simulink model "solution1_7009_newfmu"  (R2017b)
settings: Solver=FixedStepAuto  StartTime=0.0  StopTime=inf  FixedStep=0.01  RelTol=1e-3
values from neighbouring files (symbols this model uses):
  g = 9.81    [initialize_simplemodel.m]    (also in initialize_simplemodel_Trial.m; tire_friction_circle.m)
  h = 0.35    [initialize_simplemodel.m]    (also in initialize_simplemodel_Trial.m)
  lf = 1.4    [initialize_simplemodel.m]    (also in initialize_simplemodel_Trial.m)
  lr = 1.345    [initialize_simplemodel.m]    (also in initialize_simplemodel_Trial.m)
  m = 1400    [initialize_simplemodel.m]    (also in initialize_simplemodel_Trial.m = 1300; tire_friction_circle.m = 1300)
  r = 0.34    [initialize_simplemodel.m]    (also in initialize_simplemodel_Trial.m)
  tr = 1.684/2    (= 0.842)    [initialize_simplemodel.m]    (also in initialize_simplemodel_Trial.m)
  v_init = 60*5/18    (= 16.6666666667)    [initialize_simplemodel.m]    (also in initialize_simplemodel_Trial.m)
undefined symbols (not defined in the file or in its folder): DiscIntNeverNeededParam
libraries: simulink x28
(part 1 of 2)
settings Model: Creator=ashwin.ramanujam  LastModifiedBy=gandh
settings DataIOCC: SignalLogging=off

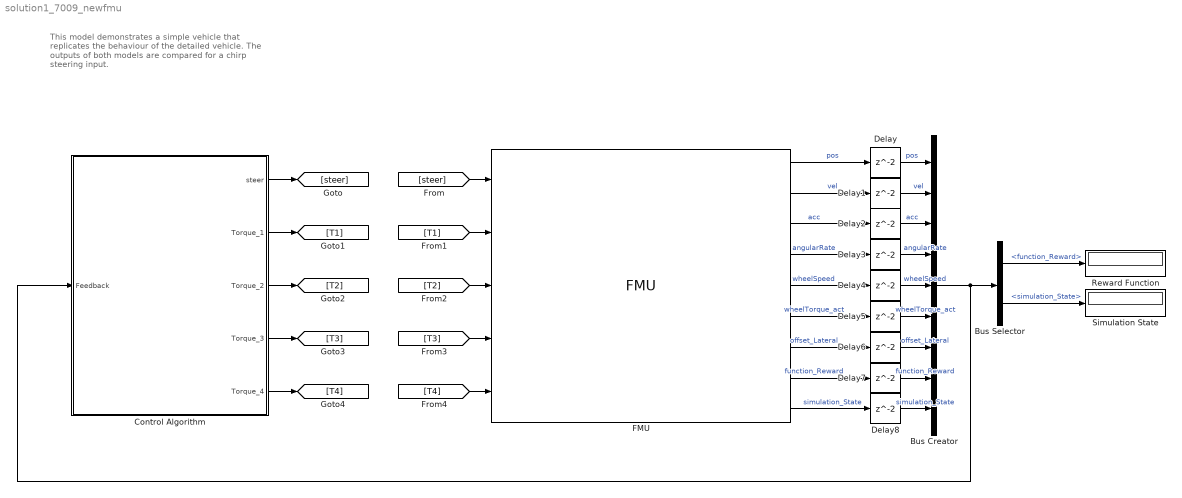
== system solution1_7009_newfmu ==
  note: This model demonstrates a simple vehicle that replicates the behaviour of the detailed vehicle. The outputs of both models are compared for a chirp steering input.
  Bus Creator : BusCreator  Inputs=9
  Bus Selector : BusSelector  OutputSignals=function_Reward,simulation_State
  Control Algorithm : Subsystem
  Delay{,1..8} (9 alike) : Delay
  FMU : FMU  FMUName=MED2018_VehicleModel_sclxversion.fmu  FMUMode=CoSimulation  FMUSampleTime=-1  mask(MED2018.VehicleModel [Co-Simulation, v2.0]){}
      mask Display:
      | disp('MED2018.VehicleModel');
      | port_label('output',1,'Position');
      | port_label('output',2,'Velocity');
      | port_label('output',3,'Acceleration');
      | port_label('output',4,'angularRate');
      | port_label('output',5,'wheelSpeed');
      | port_label('output',6,'wheelTorque_act');
      | port_label('output',7,'offset_Lateral');
      | port_label('output',8,'function_Reward');
      | port_label('output',9,'simulation_State');
      | port_label('input',1,'steering_Angle');
      | port_label('input',2,'wheelTorque_cmd_FL');
      | port_label('input',3,'wheelTorque_cmd_FR');
      | port_label('input',4,'wheelTorque_cmd_RL');
      | port_label('input',5,'wheelTorque_cmd_RR');
  Reward Function : Display
  Simulation State : Display
  wires:
  [steer] -> FMU/1
  [T4] -> FMU/5
  [T1] -> FMU/2
  [T2] -> FMU/3
  [T3] -> FMU/4
  Control Algorithm/1(steer) -> [steer]
  Control Algorithm/2(Torque_1) -> [T1]
  Control Algorithm/3(Torque_2) -> [T2]
  Control Algorithm/4(Torque_3) -> [T3]
  Control Algorithm/5(Torque_4) -> [T4]
  FMU/1 -> Delay/1  "pos"
  FMU/6 -> Delay5/1  "wheelTorque_act"
  FMU/8 -> Delay7/1  "function_Reward"
  FMU/3 -> Delay2/1  "acc"
  FMU/5 -> Delay4/1  "wheelSpeed"
  FMU/7 -> Delay6/1  "offset_Lateral"
  FMU/2 -> Delay1/1  "vel"
  FMU/4 -> Delay3/1  "angularRate"
  FMU/9 -> Delay8/1  "simulation_State"
  Bus Creator/1 -> Control Algorithm/1(Feedback), Bus Selector/1
  Bus Selector/1 -> Reward Function/1  "<function_Reward>"
  Bus Selector/2 -> Simulation State/1  "<simulation_State>"
  Delay/1 -> Bus Creator/1  "pos"
  Delay1/1 -> Bus Creator/2  "vel"
  Delay2/1 -> Bus Creator/3  "acc"
  Delay3/1 -> Bus Creator/4  "angularRate"
  Delay4/1 -> Bus Creator/5  "wheelSpeed"
  Delay5/1 -> Bus Creator/6  "wheelTorque_act"
  Delay6/1 -> Bus Creator/7  "offset_Lateral"
  Delay7/1 -> Bus Creator/8  "function_Reward"
  Delay8/1 -> Bus Creator/9  "simulation_State"

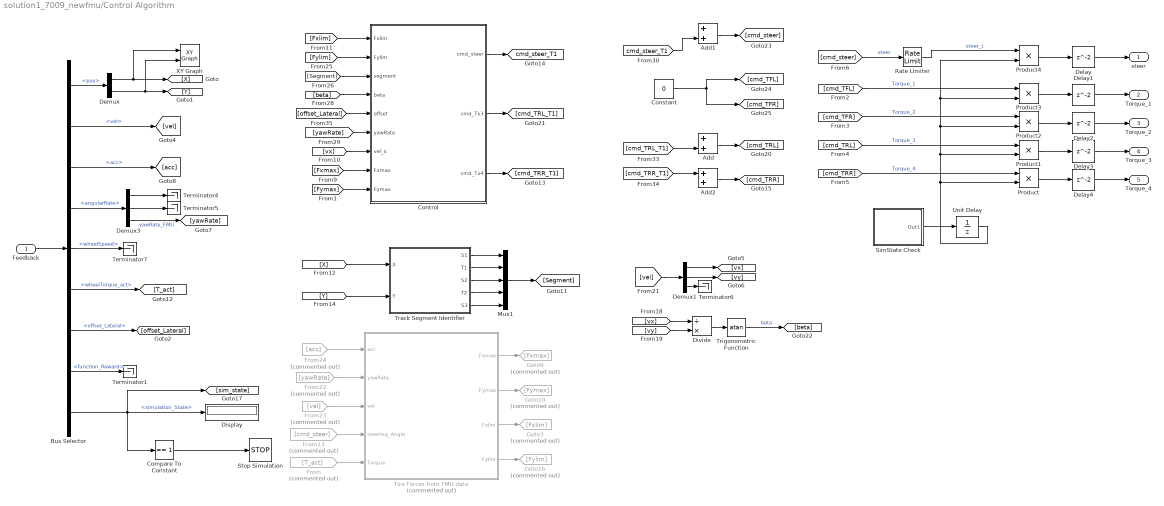
== system solution1_7009_newfmu/Control Algorithm ==
  Feedback : Inport
  Add : Sum
  Add1 : Sum
  Add2 : Sum
  Bus Selector : BusSelector  OutputSignals=pos,vel,acc,angularRate,wheelSpeed,wheelTorque_act,offset_Lateral,function_Reward,simulation_State
  Compare To Constant : simulink/Logic and Bit Operations/Compare To Constant  relop===  const=1  OutDataTypeStr=boolean
  Constant : Constant  Value=0
  Control : Subsystem  TreatAsAtomicUnit=on
  Delay{,1..4} (5 alike) : Delay
  Demux : Demux  Outputs=2
  Demux1 : Demux  Outputs=3
  Demux3 : Demux  Outputs=3
  Display : Display
  Divide : Product  Inputs=/*
  From : From  Commented=on  GotoTag=T_act
  From13 : From  Commented=on  GotoTag=cmd_steer
  From22 : From  Commented=on  GotoTag=yawRate
  From23 : From  Commented=on  GotoTag=vel
  From24 : From  Commented=on  GotoTag=acc
  Goto10 : Goto  Commented=on  GotoTag=Fymax
  Goto16 : Goto  Commented=on  GotoTag=Fylim
  Goto3 : Goto  Commented=on  GotoTag=Fxlim
  Goto9 : Goto  Commented=on  GotoTag=Fxmax
  Mux1 : Mux  Inputs=5
  Product{,1..4} (5 alike) : Product
  Rate Limiter : RateLimiter  RisingSlewLimit=500*pi/180  FallingSlewLimit=-500*pi/180  SampleTimeMode=inherited
  SimState Check : Subsystem
  Stop Simulation : Stop
  Terminator{1,4..7} (5 alike) : Terminator
  Tire Forces from FMU data : Subsystem  Commented=on  TreatAsAtomicUnit=on
  Track Segment Identifier : Subsystem
  Trigonometric Function : Trigonometry  Operator=atan
  Unit Delay : UnitDelay  SampleTime=-1
  XY Graph : simulink/Sinks/XY Graph  xmin=-5  xmax=110  ymin=-10  ymax=180  st=-1
  steer : Outport
  Torque_1 : Outport  Port=2
  Torque_2 : Outport  Port=3
  Torque_3 : Outport  Port=4
  Torque_4 : Outport  Port=5
  tag scope: cmd_steer_T1=global
  wires:
  [cmd_steer] -> Rate Limiter/1  "steer"
  Feedback/1 -> Bus Selector/1
  Bus Selector/1 -> Demux/1  "<pos>"
  Demux/2 -> XY Graph/2, [Y]
  Demux/1 -> XY Graph/1, [X]
  Bus Selector/2 -> [vel]  "<vel>"
  Bus Selector/3 -> [acc]  "<acc>"
  Demux3/1 -> Terminator4/1
  Demux3/2 -> Terminator5/1
  Bus Selector/4 -> Demux3/1  "<angularRate>"
  Bus Selector/5 -> Terminator7/1  "<wheelSpeed>"
  Bus Selector/8 -> Terminator1/1  "<function_Reward>"
  Bus Selector/9 -> Compare To Constant/1, Display/1, [sim_state]  "<simulation_State>"
  Compare To Constant/1 -> Stop Simulation/1
  From13/1 -> Tire Forces from FMU data/4(steering_Angle)
  From/1 -> Tire Forces from FMU data/5(Torque)
  Bus Selector/6 -> [T_act]  "<wheelTorque_act>"
  Bus Selector/7 -> [offset_Lateral]  "<offset_Lateral>"
  Demux3/3 -> [yawRate]  "yawRate_FMU"
  [X] -> Track Segment Identifier/1(X)
  [Y] -> Track Segment Identifier/2(Y)
  Tire Forces from FMU data/2(Fymax) -> Goto10/1
  Tire Forces from FMU data/1(Fxmax) -> Goto9/1
  Track Segment Identifier/1(S1) -> Mux1/1
  Track Segment Identifier/2(T1) -> Mux1/2
  Track Segment Identifier/3(S2) -> Mux1/3
  Track Segment Identifier/4(T2) -> Mux1/4
  Track Segment Identifier/5(S3) -> Mux1/5
  Mux1/1 -> [Segment]
  Trigonometric Function/1 -> [beta]  "beta"
  [vy] -> Divide/2
  Divide/1 -> Trigonometric Function/1
  [vx] -> Divide/1
  From23/1 -> Tire Forces from FMU data/3(vel)
  Demux1/2 -> [vy]
  Demux1/3 -> Terminator6/1
  Demux1/1 -> [vx]
  [vel] -> Demux1/1
  From22/1 -> Tire Forces from FMU data/2(yawRate)
  From24/1 -> Tire Forces from FMU data/1(acc)
  [vx] -> Control/7(vel_x)
  [Segment] -> Control/3(segment)
  [Fylim] -> Control/2(Fylim)
  [Fxlim] -> Control/1(Fxlim)
  Control/3(cmd_Tx4) -> [cmd_TRR_T1]
  Control/2(cmd_Tx3) -> [cmd_TRL_T1]
  Control/1(cmd_steer) -> [cmd_steer_T1]
  [beta] -> Control/4(beta)
  [yawRate] -> Control/6(yawRate)
  [cmd_TRL_T1] -> Add/2
  [cmd_steer_T1] -> Add1/2
  [cmd_TRR_T1] -> Add2/1
  Add2/1 -> [cmd_TRR]
  Add/1 -> [cmd_TRL]
  Add1/1 -> [cmd_steer]
  [offset_Lateral] -> Control/5(offset)
  [Fxmax] -> Control/8("Fxmax ")
  Tire Forces from FMU data/3(Fxlim) -> Goto3/1
  Tire Forces from FMU data/4(Fylim) -> Goto16/1
  [Fymax] -> Control/9(Fymax)
  Constant/1 -> [cmd_TFL], [cmd_TFR]
  Product3/1 -> Delay1/1
  Product2/1 -> Delay2/1
  Product1/1 -> Delay3/1
  Product/1 -> Delay4/1
  Product4/1 -> Delay/1
  Rate Limiter/1 -> Product4/1  "steer_c"
  [cmd_TFL] -> Product3/1  "Torque_1"
  [cmd_TFR] -> Product2/1  "Torque_2"
  [cmd_TRL] -> Product1/1  "Torque_3"
  [cmd_TRR] -> Product/1  "Torque_4"
  Unit Delay/1 -> Product1/2, Product2/2, Product3/2, Product4/2, Product/2
  SimState Check/1(Out1) -> Unit Delay/1
  Delay/1 -> steer/1
  Delay1/1 -> Torque_1/1
  Delay2/1 -> Torque_2/1
  Delay3/1 -> Torque_3/1
  Delay4/1 -> Torque_4/1

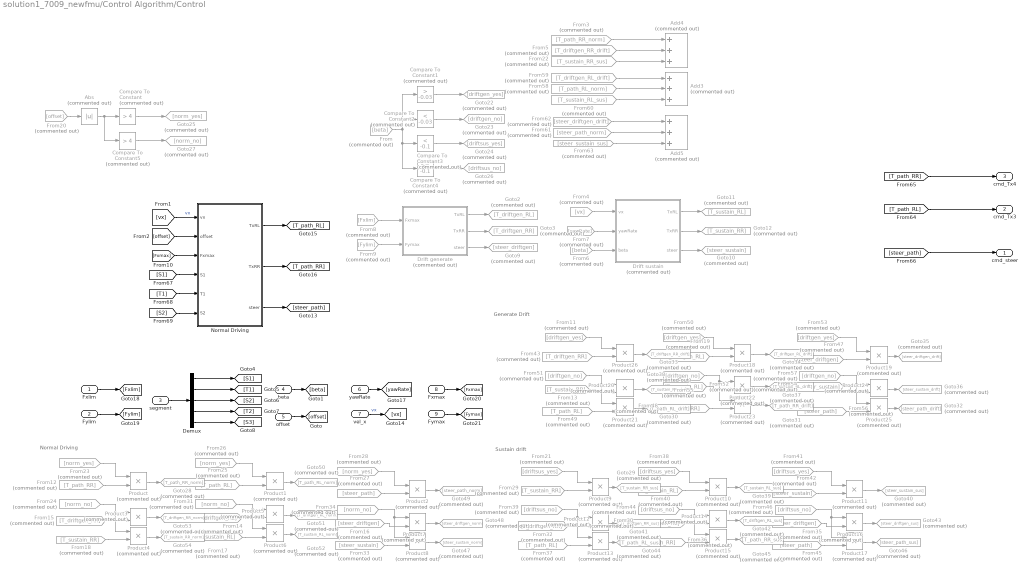
== system solution1_7009_newfmu/Control Algorithm/Control ==
  note: Generate Drift
  note: Sustain drift
  note: Normal Driving
  Fxlim : Inport
  Fylim : Inport  Port=2
  segment : Inport  Port=3
  beta : Inport  Port=4
  offset : Inport  Port=5
  yawRate : Inport  Port=6
  vel_x : Inport  Port=7
  "Fxmax " : Inport  Port=8
  Fymax : Inport  Port=9
  Abs : Abs  Commented=on
  Add3 : Sum  Commented=on  Inputs=+++
  Add4 : Sum  Commented=on  Inputs=+++
  Add5 : Sum  Commented=on  Inputs=+++
  Compare To Constant : simulink/Logic and Bit Operations/Compare To Constant  Commented=on  relop=>  const=4  OutDataTypeStr=boolean
  Compare To Constant1 : simulink/Logic and Bit Operations/Compare To Constant  Commented=on  relop=>  const=-0.03  OutDataTypeStr=boolean
  Compare To Constant2 : simulink/Logic and Bit Operations/Compare To Constant  Commented=on  relop=<  const=-0.03  OutDataTypeStr=boolean
  Compare To Constant3 : simulink/Logic and Bit Operations/Compare To Constant  Commented=on  relop=<  const=-0.1  OutDataTypeStr=boolean
  Compare To Constant4 : simulink/Logic and Bit Operations/Compare To Constant  Commented=on  relop=>=  const=-0.1  OutDataTypeStr=boolean
  Compare To Constant5 : simulink/Logic and Bit Operations/Compare To Constant  Commented=on  relop=>  const=4  OutDataTypeStr=boolean
  Demux : Demux  Outputs=5
  Drift generate : Subsystem  Commented=on
  Drift sustain : Subsystem  Commented=on
  From : From  Commented=on  GotoTag=beta
  From11 : From  Commented=on  GotoTag=driftgen_yes
  From12 : From  Commented=on  GotoTag=T_path_RR
  From13 : From  Commented=on  GotoTag=T_sustain_RR
  From14 : From  Commented=on  GotoTag=T_driftgen_RL
  From15 : From  Commented=on  GotoTag=T_driftgen_RR
  From16 : From  Commented=on  GotoTag=steer_driftgen
  From17 : From  Commented=on  GotoTag=T_sustain_RL
  From18 : From  Commented=on  GotoTag=T_sustain_RR
  From19 : From  Commented=on  GotoTag=T_driftgen_RL
  From20 : From  Commented=on  GotoTag=offset
  From21 : From  Commented=on  GotoTag=driftsus_yes
  From22 : From  Commented=on  GotoTag=T_sustain_RR_sus
  From23 : From  Commented=on  GotoTag=norm_yes
  From24 : From  Commented=on  GotoTag=norm_no
  From25 : From  Commented=on  GotoTag=T_path_RL
  From26 : From  Commented=on  GotoTag=norm_yes
  From27 : From  Commented=on  GotoTag=steer_path
  From28 : From  Commented=on  GotoTag=norm_yes
  From29 : From  Commented=on  GotoTag=T_sustain_RR
  From3 : From  Commented=on  GotoTag=T_path_RR_norm
  From30 : From  Commented=on  GotoTag=T_driftgen_RL
  From31 : From  Commented=on  GotoTag=norm_no
  From32 : From  Commented=on  GotoTag=T_driftgen_RR
  From33 : From  Commented=on  GotoTag=steer_sustain
  From34 : From  Commented=on  GotoTag=norm_no
  From35 : From  Commented=on  GotoTag=steer_driftgen
  From36 : From  Commented=on  GotoTag=T_path_RR
  From37 : From  Commented=on  GotoTag=T_path_RL
  From38 : From  Commented=on  GotoTag=driftsus_yes
  From39 : From  Commented=on  GotoTag=driftsus_no
  From4 : From  Commented=on  GotoTag=vx
  From40 : From  Commented=on  GotoTag=T_sustain_RL
  From41 : From  Commented=on  GotoTag=driftsus_yes
  From42 : From  Commented=on  GotoTag=steer_sustain
  From43 : From  Commented=on  GotoTag=T_driftgen_RR
  From44 : From  Commented=on  GotoTag=driftsus_no
  From45 : From  Commented=on  GotoTag=steer_path
  From46 : From  Commented=on  GotoTag=driftsus_no
  From47 : From  Commented=on  GotoTag=steer_driftgen
  From48 : From  Commented=on  GotoTag=T_path_RR
  From49 : From  Commented=on  GotoTag=T_path_RL
  From5 : From  Commented=on  GotoTag=T_driftgen_RR_drift
  From50 : From  Commented=on  GotoTag=driftgen_yes
  From51 : From  Commented=on  GotoTag=driftgen_no
  From52 : From  Commented=on  GotoTag=T_sustain_RL
  From53 : From  Commented=on  GotoTag=driftgen_yes
  From54 : From  Commented=on  GotoTag=steer_sustain
  From55 : From  Commented=on  GotoTag=driftgen_no
  From56 : From  Commented=on  GotoTag=steer_path
  From57 : From  Commented=on  GotoTag=driftgen_no
  From58 : From  Commented=on  GotoTag=T_path_RL_norm
  From59 : From  Commented=on  GotoTag=T_driftgen_RL_drift
  From6 : From  Commented=on  GotoTag=beta
  From60 : From  Commented=on  GotoTag=T_sustain_RL_sus
  From61 : From  Commented=on  GotoTag=steer_path_norm
  From62 : From  Commented=on  GotoTag=steer_driftgen_drift
  From63 : From  Commented=on  GotoTag=steer_sustain_sus
  From7 : From  Commented=on  GotoTag=yawRate
  From8 : From  Commented=on  GotoTag=Fxlim
  From9 : From  Commented=on  GotoTag=Fylim
  Goto10 : Goto  Commented=on  GotoTag=steer_sustain
  Goto11 : Goto  Commented=on  GotoTag=T_sustain_RL
  Goto12 : Goto  Commented=on  GotoTag=T_sustain_RR
  Goto2 : Goto  Commented=on  GotoTag=T_driftgen_RL
  Goto22 : Goto  Commented=on  GotoTag=driftgen_yes
  Goto23 : Goto  Commented=on  GotoTag=driftgen_no
  Goto24 : Goto  Commented=on  GotoTag=driftsus_yes
  Goto25 : Goto  Commented=on  GotoTag=norm_yes
  Goto26 : Goto  Commented=on  GotoTag=driftsus_no
  Goto27 : Goto  Commented=on  GotoTag=norm_no
  Goto28 : Goto  Commented=on  GotoTag=T_path_RR_norm
  Goto29 : Goto  Commented=on  GotoTag=T_sustain_RR_sus
  Goto3 : Goto  Commented=on  GotoTag=T_driftgen_RR
  Goto30 : Goto  Commented=on  GotoTag=T_path_RL_drift
  Goto31 : Goto  Commented=on  GotoTag=T_path_RR_drift
  Goto32 : Goto  Commented=on  GotoTag=steer_path_drift
  Goto33 : Goto  Commented=on  GotoTag=T_driftgen_RR_drift
  Goto34 : Goto  Commented=on  GotoTag=T_driftgen_RL_drift
  Goto35 : Goto  Commented=on  GotoTag=steer_driftgen_drift
  Goto36 : Goto  Commented=on  GotoTag=steer_sustain_drift
  Goto37 : Goto  Commented=on  GotoTag=T_sustain_RL_drift
  Goto38 : Goto  Commented=on  GotoTag=T_sustain_RR_drift
  Goto39 : Goto  Commented=on  GotoTag=T_sustain_RL_sus
  Goto40 : Goto  Commented=on  GotoTag=steer_sustain_sus
  Goto41 : Goto  Commented=on  GotoTag=T_driftgen_RR_sus
  Goto42 : Goto  Commented=on  GotoTag=T_driftgen_RL_sus
  Goto43 : Goto  Commented=on  GotoTag=steer_driftgen_sus
  Goto44 : Goto  Commented=on  GotoTag=T_path_RL_sus
  Goto45 : Goto  Commented=on  GotoTag=T_path_RR_sus
  Goto46 : Goto  Commented=on  GotoTag=steer_path_sus
  Goto47 : Goto  Commented=on  GotoTag=steer_sustain_norm
  Goto48 : Goto  Commented=on  GotoTag=steer_driftgen_norm
  Goto49 : Goto  Commented=on  GotoTag=steer_path_norm
  Goto50 : Goto  Commented=on  GotoTag=T_path_RL_norm
  Goto51 : Goto  Commented=on  GotoTag=T_driftgen_RL_norm
  Goto52 : Goto  Commented=on  GotoTag=T_sustain_RL_norm
  Goto53 : Goto  Commented=on  GotoTag=T_driftgen_RR_norm
  Goto54 : Goto  Commented=on  GotoTag=T_sustain_RR_norm
  Goto9 : Goto  Commented=on  GotoTag=steer_driftgen
  Normal Driving : Subsystem
  Product{,1..26} (27 alike) : Product  Commented=on
  cmd_steer : Outport
  cmd_Tx3 : Outport  Port=2
  cmd_Tx4 : Outport  Port=3
  wires:
  Demux/5 -> [S3]
  Demux/4 -> [T2]
  Demux/3 -> [S2]
  Demux/2 -> [T1]
  Demux/1 -> [S1]
  segment/1 -> Demux/1
  beta/1 -> [beta]
  Abs/1 -> Compare To Constant5/1, Compare To Constant/1
  offset/1 -> [offset]
  Drift generate/1(TxRL) -> Goto2/1
  Drift generate/2(TxRR) -> Goto3/1
  Drift generate/3(steer) -> Goto9/1
  Drift sustain/3(steer) -> Goto10/1
  vel_x/1 -> [vx]  "vx"
  From4/1 -> Drift sustain/1(vx)
  [vx] -> Normal Driving/1(vx)  "vx"
  [offset] -> Normal Driving/2(offset)
  Normal Driving/3(steer) -> [steer_path]
  Normal Driving/2(TxRR) -> [T_path_RR]
  Normal Driving/1(TxRL) -> [T_path_RL]
  From6/1 -> Drift sustain/3(beta)
  yawRate/1 -> [yawRate]
  From7/1 -> Drift sustain/2(yawRate)
  Drift sustain/2(TxRR) -> Goto12/1
  Drift sustain/1(TxRL) -> Goto11/1
  Fxlim/1 -> [Fxlim]
  Fylim/1 -> [Fylim]
  From8/1 -> Drift generate/1(Fxmax)
  From9/1 -> Drift generate/2(Fymax)
  "Fxmax "/1 -> [Fxmax]
  [Fxmax] -> Normal Driving/3(Fxmax)
  Fymax/1 -> [Fymax]
  From20/1 -> Abs/1
  From/1 -> Compare To Constant1/1, Compare To Constant2/1, Compare To Constant4/1, Compare To Constant3/1
  Compare To Constant2/1 -> Goto23/1
  Compare To Constant1/1 -> Goto22/1
  Compare To Constant3/1 -> Goto24/1
  Compare To Constant4/1 -> Goto26/1
  Compare To Constant/1 -> Goto25/1
  From12/1 -> Product/2
  Compare To Constant5/1 -> Goto27/1
  From23/1 -> Product/1
  From26/1 -> Product1/1
  From25/1 -> Product1/2
  From28/1 -> Product2/1
  From27/1 -> Product2/2
  From15/1 -> Product3/2
  From24/1 -> Product3/1, Product4/1
  From18/1 -> Product4/2
  From17/1 -> Product6/2
  From31/1 -> Product6/1, Product5/1
  From14/1 -> Product5/2
  From16/1 -> Product7/2
  From34/1 -> Product7/1, Product8/1
  From33/1 -> Product8/2
  From45/1 -> Product17/2
  From46/1 -> Product17/1, Product16/1
  From35/1 -> Product16/2
  From30/1 -> Product14/2
  From44/1 -> Product14/1, Product15/1
  From36/1 -> Product15/2
  From37/1 -> Product13/2
  From39/1 -> Product13/1, Product12/1
  From32/1 -> Product12/2
  From42/1 -> Product11/2
  From41/1 -> Product11/1
  From40/1 -> Product10/2
  From38/1 -> Product10/1
  From21/1 -> Product9/1
  From29/1 -> Product9/2
  From11/1 -> Product26/1
  From50/1 -> Product18/1
  From53/1 -> Product19/1
  From51/1 -> Product20/1, Product21/1
  From49/1 -> Product21/2
  From48/1 -> Product23/2
  From55/1 -> Product23/1, Product22/1
  From57/1 -> Product24/1, Product25/1
  From56/1 -> Product25/2
  From43/1 -> Product26/2
  From13/1 -> Product20/2
  From19/1 -> Product18/2
  From52/1 -> Product22/2
  From47/1 -> Product19/2
  From54/1 -> Product24/2
  Product/1 -> Goto28/1
  Product26/1 -> Goto33/1
  Product9/1 -> Goto29/1
  Product20/1 -> Goto38/1
  Product21/1 -> Goto30/1
  Product18/1 -> Goto34/1
  Product22/1 -> Goto37/1
  Product23/1 -> Goto31/1
  Product25/1 -> Goto32/1
  Product24/1 -> Goto36/1
  Product19/1 -> Goto35/1
  Product11/1 -> Goto40/1
  Product16/1 -> Goto43/1
  Product17/1 -> Goto46/1
  Product10/1 -> Goto39/1
  Product14/1 -> Goto42/1
  Product15/1 -> Goto45/1
  Product12/1 -> Goto41/1
  Product13/1 -> Goto44/1
  Product8/1 -> Goto47/1
  Product7/1 -> Goto48/1
  Product2/1 -> Goto49/1
  Product1/1 -> Goto50/1
  Product5/1 -> Goto51/1
  Product6/1 -> Goto52/1
  Product3/1 -> Goto53/1
  Product4/1 -> Goto54/1
  From22/1 -> Add4/3
  From5/1 -> Add4/2
  From3/1 -> Add4/1
  From59/1 -> Add3/1
  From58/1 -> Add3/2
  From60/1 -> Add3/3
  From62/1 -> Add5/1
  From61/1 -> Add5/2
  From63/1 -> Add5/3
  [steer_path] -> cmd_steer/1
  [S1] -> Normal Driving/4(S1)
  [T1] -> Normal Driving/5(T1)
  [S2] -> Normal Driving/6(S2)
  [T_path_RR] -> cmd_Tx4/1
  [T_path_RL] -> cmd_Tx3/1

== system solution1_7009_newfmu/Control Algorithm/SimState Check ==
  Compare To Constant : simulink/Logic and Bit Operations/Compare To Constant  relop===  const=-1  OutDataTypeStr=boolean
  Constant1 : Constant
  Constant2 : Constant  Value=0
  Switch : Switch  Criteria=u2 > Threshold
  Out1 : Outport
  wires:
  Constant1/1 -> Switch/3
  Compare To Constant/1 -> Switch/2
  Switch/1 -> Out1/1
  [sim_state] -> Compare To Constant/1
  Constant2/1 -> Switch/1

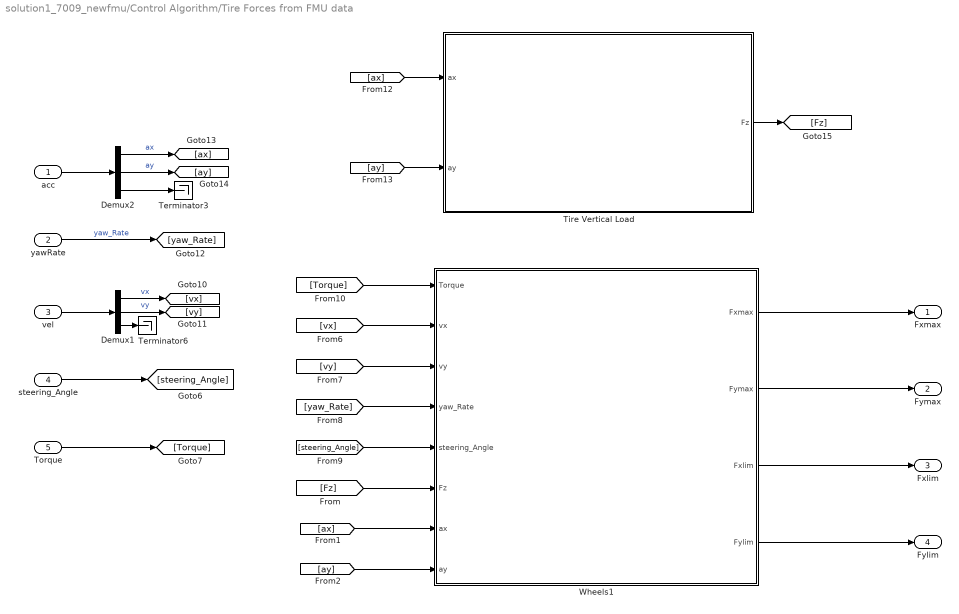
== system solution1_7009_newfmu/Control Algorithm/Tire Forces from FMU data ==
  acc : Inport
  yawRate : Inport  Port=2
  vel : Inport  Port=3
  steering_Angle : Inport  Port=4
  Torque : Inport  Port=5
  Demux1 : Demux  Outputs=3
  Demux2 : Demux  Outputs=3
  Terminator3 : Terminator
  Terminator6 : Terminator
  Tire Vertical Load : MATLAB Function  TreatAsAtomicUnit=on
  Wheels1 : Subsystem  Priority=0
  Fxmax : Outport
  Fymax : Outport  Port=2
  Fxlim : Outport  Port=3
  Fylim : Outport  Port=4
  wires:
  [vy] -> Wheels1/3(vy)
  [Torque] -> Wheels1/1(Torque)
  [yaw_Rate] -> Wheels1/4(yaw_Rate)
  [vx] -> Wheels1/2(vx)
  [Fz] -> Wheels1/6(Fz)
  [steering_Angle] -> Wheels1/5(steering_Angle)
  Torque/1 -> [Torque]
  Wheels1/3(Fxlim) -> Fxlim/1
  Wheels1/4(Fylim) -> Fylim/1
  Wheels1/1(Fxmax) -> Fxmax/1
  Wheels1/2(Fymax) -> Fymax/1
  Demux1/2 -> [vy]  "vy"
  Demux1/3 -> Terminator6/1
  Demux1/1 -> [vx]  "vx"
  vel/1 -> Demux1/1
  yawRate/1 -> [yaw_Rate]  "yaw_Rate"
  Demux2/1 -> [ax]  "ax"
  Demux2/2 -> [ay]  "ay"
  Demux2/3 -> Terminator3/1
  acc/1 -> Demux2/1
  [ay] -> Tire Vertical Load/2(ay)
  [ax] -> Tire Vertical Load/1(ax)
  Tire Vertical Load/1(Fz) -> [Fz]
  [ax] -> Wheels1/7(ax)
  [ay] -> Wheels1/8(ay)
  steering_Angle/1 -> [steering_Angle]

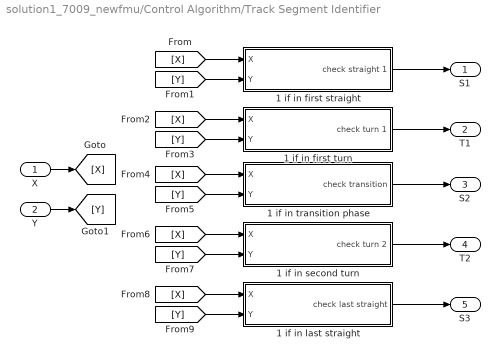
== system solution1_7009_newfmu/Control Algorithm/Track Segment Identifier ==
  X : Inport
  Y : Inport  Port=2
  1 if in first straight : Subsystem
  1 if in first turn : Subsystem
  1 if in last straight : Subsystem
  1 if in second turn : Subsystem
  1 if in transition phase : Subsystem
  S1 : Outport
  T1 : Outport  Port=2
  S2 : Outport  Port=3
  T2 : Outport  Port=4
  S3 : Outport  Port=5
  wires:
  1 if in first turn/1(check turn 1) -> T1/1
  1 if in second turn/1(check turn 2) -> T2/1
  1 if in last straight/1(check last straight) -> S3/1
  1 if in first straight/1(check straight 1) -> S1/1
  1 if in transition phase/1(check transition) -> S2/1
  X/1 -> [X]
  Y/1 -> [Y]
  [X] -> 1 if in first straight/1(X)
  [Y] -> 1 if in first straight/2(Y)
  [Y] -> 1 if in first turn/2(Y)
  [X] -> 1 if in first turn/1(X)
  [X] -> 1 if in transition phase/1(X)
  [Y] -> 1 if in transition phase/2(Y)
  [Y] -> 1 if in second turn/2(Y)
  [X] -> 1 if in second turn/1(X)
  [X] -> 1 if in last straight/1(X)
  [Y] -> 1 if in last straight/2(Y)

== system solution1_7009_newfmu/Control Algorithm/Control/Drift generate ==
  note: Big turn in
  Fxmax : Inport
  Fymax : Inport  Port=2
  Constant1 : Constant  Value=0
  Discrete PID Controller1 : simulink/Continuous/PID Controller  Controller=PID  TimeDomain=Discrete-time  SampleTime=-1  IntegratorMethod=Forward Euler  FilterMethod=Forward Euler  Form=Parallel  UseFilter=on  ControllerParametersSource=internal  P=2  I=0  D=0.1  N=100  InitialConditionSource=internal  InitialConditionForIntegrator=0  InitialConditionForFilter=0  ExternalReset=none  LimitOutput=off  UpperSaturationLimit=inf  LowerSaturationLimit=-inf  LinearizeAsGain=off  AntiWindupMode=none  Kb=1  TrackingMode=off  Kt=1  PParamMin=[]  PParamMax=[]  IParamMin=[]  IParamMax=[]  DParamMin=[]  DParamMax=[]  NParamMin=[]  NParamMax=[]  KbParamMin=[]  KbParamMax=[]  KtParamMin=[]  KtParamMax=[]  POutMin=[]  POutMax=[]  IOutMin=[]  IOutMax=[]  DOutMin=[]  DOutMax=[]  NOutMin=[]  NOutMax=[]  KbOutMin=[]  KbOutMax=[]  KtOutMin=[]  KtOutMax=[]  IntegratorOutMin=[]  IntegratorOutMax=[]  FilterOutMin=[]  FilterOutMax=[]  SumOutMin=[]  SumOutMax=[]  SumI1OutMin=[]  SumI1OutMax=[]  SumI2OutMin=[]  SumI2OutMax=[]  SumI3OutMin=[]  SumI3OutMax=[]  SumDOutMin=[]  SumDOutMax=[]  SaturationOutMin=[]  SaturationOutMax=[]  IntegratorContinuousStateAttributes=''  IntegratorStateMustResolveToSignalObject=off  IntegratorRTWStateStorageClass=Auto  FilterContinuousStateAttributes=''  FilterStateMustResolveToSignalObject=off  FilterRTWStateStorageClass=Auto  DifferentiatorICPrevScaledInput=0  DifferentiatorOutMin=[]  DifferentiatorOutMax=[]  InitialConditionSetting=State (most efficient)  FilterDiffOutCoefMin=[]  FilterDiffOutCoefMax=[]  SumDenOutMin=[]  SumDenOutMax=[]  SumNumOutMin=[]  SumNumOutMax=[]  ReciprocalOutMin=[]  ReciprocalOutMax=[]  DivideOutMin=[]  DivideOutMax=[]  TunerSelectOption=Transfer Function Based (PID Tuner App)
  Max wheel force : Subsystem
  Subtract1 : Sum  Inputs=+-
  TxRL : Outport
  TxRR : Outport  Port=2
  steer : Outport  Port=3
  wires:
  Max wheel force/2(TxRR) -> TxRR/1
  Fxmax/1 -> Max wheel force/1(Fxmax)
  Fymax/1 -> Max wheel force/2(Fymax)
  Constant1/1 -> Subtract1/1
  Subtract1/1 -> Discrete PID Controller1/1  "offset_error"
  [offset] -> Subtract1/2
  Max wheel force/1(TxRL) -> TxRL/1
  Discrete PID Controller1/1 -> steer/1  "steer"

== system solution1_7009_newfmu/Control Algorithm/Control/Drift sustain ==
  vx : Inport
  yawRate : Inport  Port=2
  beta : Inport  Port=3
  Constant : Constant  Value=0
  Discrete PID Controller : simulink/Continuous/PID Controller  Controller=PID  TimeDomain=Discrete-time  SampleTime=-1  IntegratorMethod=Forward Euler  FilterMethod=Forward Euler  Form=Parallel  UseFilter=on  ControllerParametersSource=internal  P=1  I=0  D=0.1  N=100  InitialConditionSource=internal  InitialConditionForIntegrator=0  InitialConditionForFilter=0  ExternalReset=none  LimitOutput=off  UpperSaturationLimit=inf  LowerSaturationLimit=-inf  LinearizeAsGain=off  AntiWindupMode=none  Kb=1  TrackingMode=off  Kt=1  PParamMin=[]  PParamMax=[]  IParamMin=[]  IParamMax=[]  DParamMin=[]  DParamMax=[]  NParamMin=[]  NParamMax=[]  KbParamMin=[]  KbParamMax=[]  KtParamMin=[]  KtParamMax=[]  POutMin=[]  POutMax=[]  IOutMin=[]  IOutMax=[]  DOutMin=[]  DOutMax=[]  NOutMin=[]  NOutMax=[]  KbOutMin=[]  KbOutMax=[]  KtOutMin=[]  KtOutMax=[]  IntegratorOutMin=[]  IntegratorOutMax=[]  FilterOutMin=[]  FilterOutMax=[]  SumOutMin=[]  SumOutMax=[]  SumI1OutMin=[]  SumI1OutMax=[]  SumI2OutMin=[]  SumI2OutMax=[]  SumI3OutMin=[]  SumI3OutMax=[]  SumDOutMin=[]  SumDOutMax=[]  SaturationOutMin=[]  SaturationOutMax=[]  IntegratorContinuousStateAttributes=''  IntegratorStateMustResolveToSignalObject=off  IntegratorRTWStateStorageClass=Auto  FilterContinuousStateAttributes=''  FilterStateMustResolveToSignalObject=off  FilterRTWStateStorageClass=Auto  DifferentiatorICPrevScaledInput=0  DifferentiatorOutMin=[]  DifferentiatorOutMax=[]  InitialConditionSetting=State (most efficient)  FilterDiffOutCoefMin=[]  FilterDiffOutCoefMax=[]  SumDenOutMin=[]  SumDenOutMax=[]  SumNumOutMin=[]  SumNumOutMax=[]  ReciprocalOutMin=[]  ReciprocalOutMax=[]  DivideOutMin=[]  DivideOutMax=[]  TunerSelectOption=Transfer Function Based (PID Tuner App)
  Discrete PID Controller5 : simulink/Continuous/PID Controller  Controller=PID  TimeDomain=Discrete-time  SampleTime=-1  IntegratorMethod=Forward Euler  FilterMethod=Forward Euler  Form=Parallel  UseFilter=off  ControllerParametersSource=internal  P=100  I=0  D=1  N=100  InitialConditionSource=internal  InitialConditionForIntegrator=0  InitialConditionForFilter=0  ExternalReset=none  LimitOutput=off  UpperSaturationLimit=inf  LowerSaturationLimit=-inf  LinearizeAsGain=off  AntiWindupMode=none  Kb=1  TrackingMode=off  Kt=1  PParamMin=[]  PParamMax=[]  IParamMin=[]  IParamMax=[]  DParamMin=[]  DParamMax=[]  NParamMin=[]  NParamMax=[]  KbParamMin=[]  KbParamMax=[]  KtParamMin=[]  KtParamMax=[]  POutMin=[]  POutMax=[]  IOutMin=[]  IOutMax=[]  DOutMin=[]  DOutMax=[]  NOutMin=[]  NOutMax=[]  KbOutMin=[]  KbOutMax=[]  KtOutMin=[]  KtOutMax=[]  IntegratorOutMin=[]  IntegratorOutMax=[]  FilterOutMin=[]  FilterOutMax=[]  SumOutMin=[]  SumOutMax=[]  SumI1OutMin=[]  SumI1OutMax=[]  SumI2OutMin=[]  SumI2OutMax=[]  SumI3OutMin=[]  SumI3OutMax=[]  SumDOutMin=[]  SumDOutMax=[]  SaturationOutMin=[]  SaturationOutMax=[]  IntegratorContinuousStateAttributes=''  IntegratorStateMustResolveToSignalObject=off  IntegratorRTWStateStorageClass=Auto  FilterContinuousStateAttributes=''  FilterStateMustResolveToSignalObject=off  FilterRTWStateStorageClass=Auto  DifferentiatorICPrevScaledInput=0  DifferentiatorOutMin=[]  DifferentiatorOutMax=[]  InitialConditionSetting=State (most efficient)  FilterDiffOutCoefMin=[]  FilterDiffOutCoefMax=[]  SumDenOutMin=[]  SumDenOutMax=[]  SumNumOutMin=[]  SumNumOutMax=[]  ReciprocalOutMin=[]  ReciprocalOutMax=[]  DivideOutMin=[]  DivideOutMax=[]  TunerSelectOption=Transfer Function Based (PID Tuner App)
  Discrete-Time Integrator : DiscreteIntegrator  InitialConditionSetting=State (most efficient)  SampleTime=-1  ICPrevOutput=DiscIntNeverNeededParam  ICPrevScaledInput=DiscIntNeverNeededParam
  Product : Product
  Subtract : Sum  Inputs=+-
  Subtract5 : Sum  Inputs=+-
  Trigonometric Function : Trigonometry  Operator=cos
  curve velocity : Constant  Value=15
  TxRL : Outport
  TxRR : Outport  Port=2
  steer : Outport  Port=3
  wires:
  beta/1 -> Trigonometric Function/1
  vx/1 -> Product/1
  curve velocity/1 -> Subtract5/1
  Trigonometric Function/1 -> Product/2
  Subtract5/1 -> Discrete PID Controller5/1  "velocity_error"
  Product/1 -> Subtract5/2
  Discrete PID Controller5/1 -> TxRR/1, TxRL/1  "cmd_Tx"
  Discrete-Time Integrator/1 -> Subtract/2
  Discrete PID Controller/1 -> steer/1
  yawRate/1 -> Discrete-Time Integrator/1
  Constant/1 -> Subtract/1
  Subtract/1 -> Discrete PID Controller/1  "moment_error"

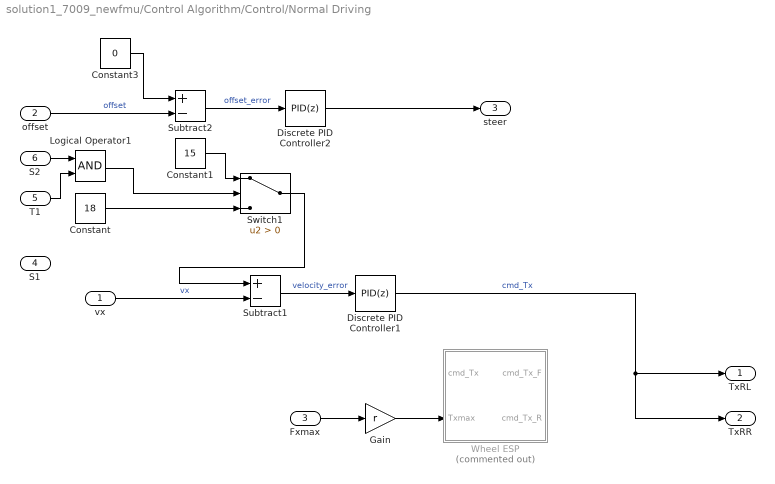
== system solution1_7009_newfmu/Control Algorithm/Control/Normal Driving ==
  vx : Inport
  offset : Inport  Port=2
  Fxmax : Inport  Port=3
  S1 : Inport  Port=4
  T1 : Inport  Port=5
  S2 : Inport  Port=6
  Constant : Constant  Value=18
  Constant1 : Constant  Value=15
  Constant3 : Constant  Value=0
  Discrete PID Controller1 : simulink/Continuous/PID Controller  Controller=PID  TimeDomain=Discrete-time  SampleTime=-1  IntegratorMethod=Forward Euler  FilterMethod=Forward Euler  Form=Parallel  UseFilter=off  ControllerParametersSource=internal  P=100  I=0  D=1  N=100  InitialConditionSource=internal  InitialConditionForIntegrator=0  InitialConditionForFilter=0  ExternalReset=none  LimitOutput=off  UpperSaturationLimit=inf  LowerSaturationLimit=-inf  LinearizeAsGain=off  AntiWindupMode=none  Kb=1  TrackingMode=off  Kt=1  PParamMin=[]  PParamMax=[]  IParamMin=[]  IParamMax=[]  DParamMin=[]  DParamMax=[]  NParamMin=[]  NParamMax=[]  KbParamMin=[]  KbParamMax=[]  KtParamMin=[]  KtParamMax=[]  POutMin=[]  POutMax=[]  IOutMin=[]  IOutMax=[]  DOutMin=[]  DOutMax=[]  NOutMin=[]  NOutMax=[]  KbOutMin=[]  KbOutMax=[]  KtOutMin=[]  KtOutMax=[]  IntegratorOutMin=[]  IntegratorOutMax=[]  FilterOutMin=[]  FilterOutMax=[]  SumOutMin=[]  SumOutMax=[]  SumI1OutMin=[]  SumI1OutMax=[]  SumI2OutMin=[]  SumI2OutMax=[]  SumI3OutMin=[]  SumI3OutMax=[]  SumDOutMin=[]  SumDOutMax=[]  SaturationOutMin=[]  SaturationOutMax=[]  IntegratorContinuousStateAttributes=''  IntegratorStateMustResolveToSignalObject=off  IntegratorRTWStateStorageClass=Auto  FilterContinuousStateAttributes=''  FilterStateMustResolveToSignalObject=off  FilterRTWStateStorageClass=Auto  DifferentiatorICPrevScaledInput=0  DifferentiatorOutMin=[]  DifferentiatorOutMax=[]  InitialConditionSetting=State (most efficient)  FilterDiffOutCoefMin=[]  FilterDiffOutCoefMax=[]  SumDenOutMin=[]  SumDenOutMax=[]  SumNumOutMin=[]  SumNumOutMax=[]  ReciprocalOutMin=[]  ReciprocalOutMax=[]  DivideOutMin=[]  DivideOutMax=[]  TunerSelectOption=Transfer Function Based (PID Tuner App)
  Discrete PID Controller2 : simulink/Continuous/PID Controller  Controller=PID  TimeDomain=Discrete-time  SampleTime=-1  IntegratorMethod=Forward Euler  FilterMethod=Forward Euler  Form=Parallel  UseFilter=on  ControllerParametersSource=internal  P=1  I=0  D=1  N=100  InitialConditionSource=internal  InitialConditionForIntegrator=0  InitialConditionForFilter=0  ExternalReset=none  LimitOutput=off  UpperSaturationLimit=inf  LowerSaturationLimit=-inf  LinearizeAsGain=off  AntiWindupMode=none  Kb=1  TrackingMode=off  Kt=1  PParamMin=[]  PParamMax=[]  IParamMin=[]  IParamMax=[]  DParamMin=[]  DParamMax=[]  NParamMin=[]  NParamMax=[]  KbParamMin=[]  KbParamMax=[]  KtParamMin=[]  KtParamMax=[]  POutMin=[]  POutMax=[]  IOutMin=[]  IOutMax=[]  DOutMin=[]  DOutMax=[]  NOutMin=[]  NOutMax=[]  KbOutMin=[]  KbOutMax=[]  KtOutMin=[]  KtOutMax=[]  IntegratorOutMin=[]  IntegratorOutMax=[]  FilterOutMin=[]  FilterOutMax=[]  SumOutMin=[]  SumOutMax=[]  SumI1OutMin=[]  SumI1OutMax=[]  SumI2OutMin=[]  SumI2OutMax=[]  SumI3OutMin=[]  SumI3OutMax=[]  SumDOutMin=[]  SumDOutMax=[]  SaturationOutMin=[]  SaturationOutMax=[]  IntegratorContinuousStateAttributes=''  IntegratorStateMustResolveToSignalObject=off  IntegratorRTWStateStorageClass=Auto  FilterContinuousStateAttributes=''  FilterStateMustResolveToSignalObject=off  FilterRTWStateStorageClass=Auto  DifferentiatorICPrevScaledInput=0  DifferentiatorOutMin=[]  DifferentiatorOutMax=[]  InitialConditionSetting=State (most efficient)  FilterDiffOutCoefMin=[]  FilterDiffOutCoefMax=[]  SumDenOutMin=[]  SumDenOutMax=[]  SumNumOutMin=[]  SumNumOutMax=[]  ReciprocalOutMin=[]  ReciprocalOutMax=[]  DivideOutMin=[]  DivideOutMax=[]  TunerSelectOption=Transfer Function Based (PID Tuner App)
  Gain : Gain  Gain=r
  Logical Operator1 : Logic  AllPortsSameDT=off  OutDataTypeStr=boolean
  Subtract1 : Sum  Inputs=+-
  Subtract2 : Sum  Inputs=+-
  Switch1 : Switch  Criteria=u2 > Threshold
  Wheel ESP : Subsystem  Commented=on
  TxRL : Outport
  TxRR : Outport  Port=2
  steer : Outport  Port=3
  wires:
  Constant3/1 -> Subtract2/1
  offset/1 -> Subtract2/2  "offset"
  Discrete PID Controller2/1 -> steer/1
  Subtract2/1 -> Discrete PID Controller2/1  "offset_error"
  Fxmax/1 -> Gain/1
  Gain/1 -> Wheel ESP/2(Txmax)
  Subtract1/1 -> Discrete PID Controller1/1  "velocity_error"
  vx/1 -> Subtract1/2  "vx"
  T1/1 -> Logical Operator1/2
  Constant/1 -> Switch1/3
  Constant1/1 -> Switch1/1
  S2/1 -> Logical Operator1/1
  Logical Operator1/1 -> Switch1/2
  Switch1/1 -> Subtract1/1
  Discrete PID Controller1/1 -> TxRR/1, TxRL/1  "cmd_Tx"

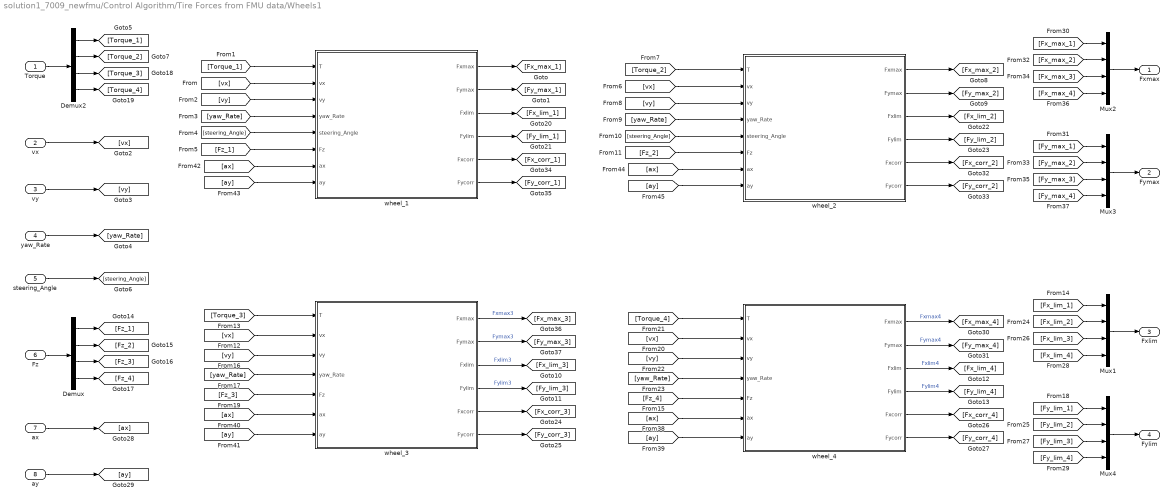
== system solution1_7009_newfmu/Control Algorithm/Tire Forces from FMU data/Wheels1 ==
  Torque : Inport
  vx : Inport  Port=2
  vy : Inport  Port=3
  yaw_Rate : Inport  Port=4
  steering_Angle : Inport  Port=5
  Fz : Inport  Port=6
  ax : Inport  Port=7
  ay : Inport  Port=8
  Demux : Demux
  Demux2 : Demux
  Mux{1..4} (4 alike) : Mux
  wheel_1 : Subsystem
  wheel_2 : Subsystem
  wheel_3 : Subsystem
  wheel_4 : Subsystem
  Fxmax : Outport
  Fymax : Outport  Port=2
  Fxlim : Outport  Port=3
  Fylim : Outport  Port=4
  wires:
  vx/1 -> [vx]
  vy/1 -> [vy]
  yaw_Rate/1 -> [yaw_Rate]
  [vx] -> wheel_1/2(vx)
  wheel_1/1(Fxmax) -> [Fx_max_1]
  wheel_1/2(Fymax) -> [Fy_max_1]
  [steering_Angle] -> wheel_1/5(steering_Angle)
  [yaw_Rate] -> wheel_1/4(yaw_Rate)
  [vy] -> wheel_1/3(vy)
  [Torque_1] -> wheel_1/1(T)
  wheel_2/1(Fxmax) -> [Fx_max_2]
  wheel_2/2(Fymax) -> [Fy_max_2]
  [yaw_Rate] -> wheel_2/4(yaw_Rate)
  [vy] -> wheel_2/3(vy)
  [steering_Angle] -> wheel_2/5(steering_Angle)
  [vx] -> wheel_2/2(vx)
  [yaw_Rate] -> wheel_3/4(yaw_Rate)
  [vy] -> wheel_4/3(vy)
  [yaw_Rate] -> wheel_4/4(yaw_Rate)
  [vx] -> wheel_4/2(vx)
  [vy] -> wheel_3/3(vy)
  [vx] -> wheel_3/2(vx)
  Demux/1 -> [Fz_1]
  Demux/2 -> [Fz_2]
  Demux/3 -> [Fz_3]
  Demux/4 -> [Fz_4]
  [Fz_1] -> wheel_1/6(Fz)
  [Fz_3] -> wheel_3/5(Fz)
  [Fz_4] -> wheel_4/5(Fz)
  [Fz_2] -> wheel_2/6(Fz)
  Fz/1 -> Demux/1
  [Torque_3] -> wheel_3/1(T)
  [Torque_2] -> wheel_2/1(T)
  [Torque_4] -> wheel_4/1(T)
  Demux2/4 -> [Torque_4]
  Demux2/3 -> [Torque_3]
  Demux2/1 -> [Torque_1]
  Torque/1 -> Demux2/1
  Demux2/2 -> [Torque_2]
  wheel_1/4(Fylim) -> [Fy_lim_1]
  wheel_2/3(Fxlim) -> [Fx_lim_2]
  wheel_2/4(Fylim) -> [Fy_lim_2]
  wheel_1/3(Fxlim) -> [Fx_lim_1]
  [Fx_max_4] -> Mux2/4
  [Fy_max_1] -> Mux3/1
  [Fy_max_4] -> Mux3/4
  [Fy_max_2] -> Mux3/2
  [Fx_max_3] -> Mux2/3
  Mux3/1 -> Fymax/1
  [Fx_max_2] -> Mux2/2
  Mux2/1 -> Fxmax/1
  [Fx_max_1] -> Mux2/1
  [Fy_max_3] -> Mux3/3
  steering_Angle/1 -> [steering_Angle]
  Mux1/1 -> Fxlim/1
  Mux4/1 -> Fylim/1
  ay/1 -> [ay]
  ax/1 -> [ax]
  [ax] -> wheel_4/6(ax)
  [ay] -> wheel_4/7(ay)
  [ay] -> wheel_3/7(ay)
  [ax] -> wheel_3/6(ax)
  [ax] -> wheel_1/7(ax)
  [ay] -> wheel_1/8(ay)
  [ay] -> wheel_2/8(ay)
  [ax] -> wheel_2/7(ax)
  wheel_2/6(Fycorr) -> [Fy_corr_2]
  wheel_2/5(Fxcorr) -> [Fx_corr_2]
  wheel_1/5(Fxcorr) -> [Fx_corr_1]
  wheel_1/6(Fycorr) -> [Fy_corr_1]
  wheel_3/5(Fxcorr) -> [Fx_corr_3]
  wheel_3/2(Fymax) -> [Fy_max_3]  "Fymax3"
  wheel_3/4(Fylim) -> [Fy_lim_3]  "Fylim3"
  wheel_3/3(Fxlim) -> [Fx_lim_3]  "Fxlim3"
  wheel_3/6(Fycorr) -> [Fy_corr_3]
  wheel_3/1(Fxmax) -> [Fx_max_3]  "Fxmax3"
  wheel_4/5(Fxcorr) -> [Fx_corr_4]
  wheel_4/2(Fymax) -> [Fy_max_4]  "Fymax4"
  wheel_4/4(Fylim) -> [Fy_lim_4]  "Fylim4"
  wheel_4/3(Fxlim) -> [Fx_lim_4]  "Fxlim4"
  wheel_4/6(Fycorr) -> [Fy_corr_4]
  wheel_4/1(Fxmax) -> [Fx_max_4]  "Fxmax4"
  [Fx_lim_1] -> Mux1/1
  [Fy_lim_1] -> Mux4/1
  [Fx_lim_2] -> Mux1/2
  [Fy_lim_2] -> Mux4/2
  [Fx_lim_3] -> Mux1/3
  [Fy_lim_3] -> Mux4/3
  [Fx_lim_4] -> Mux1/4
  [Fy_lim_4] -> Mux4/4

== system solution1_7009_newfmu/Control Algorithm/Track Segment Identifier/1 if in first straight ==
  X : Inport
  Y : Inport  Port=2
  Check Dynamic Range : simulink/Model Verification/Check  Dynamic Range  Description=min < u < max  enabled=off  stopWhenAssertionFail=off  export=on  icon=graphic
      settings: SourceProductName=Simulink  SourceProductBaseCode=SL
  Check Dynamic Range1 : simulink/Model Verification/Check  Dynamic Range  Description=min < u < max  enabled=off  stopWhenAssertionFail=off  export=on  icon=graphic
      settings: SourceProductName=Simulink  SourceProductBaseCode=SL
  Constant : Constant  Value=50
  Constant1 : Constant  Value=0
  Constant2 : Constant  Value=6
  Constant3 : Constant  Value=-6
  Logical Operator : Logic  AllPortsSameDT=off  OutDataTypeStr=boolean
  check straight 1 : Outport
  wires:
  Y/1 -> Check Dynamic Range1/3
  Check Dynamic Range1/1 -> Logical Operator/2
  Constant1/1 -> Check Dynamic Range/2
  X/1 -> Check Dynamic Range/3
  Check Dynamic Range/1 -> Logical Operator/1
  Constant3/1 -> Check Dynamic Range1/2
  Constant2/1 -> Check Dynamic Range1/1
  Logical Operator/1 -> check straight 1/1
  Constant/1 -> Check Dynamic Range/1

== system solution1_7009_newfmu/Control Algorithm/Track Segment Identifier/1 if in first turn ==
  X : Inport
  Y : Inport  Port=2
  Check Dynamic Range : simulink/Model Verification/Check  Dynamic Range  Description=min < u < max  enabled=off  stopWhenAssertionFail=off  export=on  icon=graphic
      settings: SourceProductName=Simulink  SourceProductBaseCode=SL
  Check Dynamic Range1 : simulink/Model Verification/Check  Dynamic Range  Description=min < u < max  enabled=off  stopWhenAssertionFail=off  export=on  icon=graphic
      settings: SourceProductName=Simulink  SourceProductBaseCode=SL
  Constant : Constant  Value=106
  Constant1 : Constant  Value=50
  Constant2 : Constant  Value=106
  Constant3 : Constant  Value=-6
  Logical Operator : Logic  AllPortsSameDT=off  OutDataTypeStr=boolean
  check turn 1 : Outport
  wires:
  Constant/1 -> Check Dynamic Range/1
  Logical Operator/1 -> check turn 1/1
  Constant2/1 -> Check Dynamic Range1/1
  Constant3/1 -> Check Dynamic Range1/2
  Check Dynamic Range/1 -> Logical Operator/1
  X/1 -> Check Dynamic Range/3
  Constant1/1 -> Check Dynamic Range/2
  Check Dynamic Range1/1 -> Logical Operator/2
  Y/1 -> Check Dynamic Range1/3

== system solution1_7009_newfmu/Control Algorithm/Track Segment Identifier/1 if in last straight ==
  X : Inport
  Y : Inport  Port=2
  Check Dynamic Range : simulink/Model Verification/Check  Dynamic Range  Description=min < u < max  enabled=off  stopWhenAssertionFail=off  export=on  icon=graphic
      settings: SourceProductName=Simulink  SourceProductBaseCode=SL
  Check Dynamic Range1 : simulink/Model Verification/Check  Dynamic Range  Description=min < u < max  enabled=off  stopWhenAssertionFail=off  export=on  icon=graphic
      settings: SourceProductName=Simulink  SourceProductBaseCode=SL
  Constant : Constant  Value=120
  Constant1 : Constant  Value=50
  Constant2 : Constant  Value=176
  Constant3 : Constant  Value=164
  Logical Operator : Logic  AllPortsSameDT=off  OutDataTypeStr=boolean
  check last straight : Outport
  wires:
  Y/1 -> Check Dynamic Range1/3
  Check Dynamic Range1/1 -> Logical Operator/2
  Constant1/1 -> Check Dynamic Range/2
  X/1 -> Check Dynamic Range/3
  Check Dynamic Range/1 -> Logical Operator/1
  Constant3/1 -> Check Dynamic Range1/2
  Constant2/1 -> Check Dynamic Range1/1
  Logical Operator/1 -> check last straight/1
  Constant/1 -> Check Dynamic Range/1

== system solution1_7009_newfmu/Control Algorithm/Track Segment Identifier/1 if in second turn ==
  X : Inport
  Y : Inport  Port=2
  Check Dynamic Range : simulink/Model Verification/Check  Dynamic Range  Description=min < u < max  enabled=off  stopWhenAssertionFail=off  export=on  icon=graphic
      settings: SourceProductName=Simulink  SourceProductBaseCode=SL
  Check Dynamic Range1 : simulink/Model Verification/Check  Dynamic Range  Description=min < u < max  enabled=off  stopWhenAssertionFail=off  export=on  icon=graphic
      settings: SourceProductName=Simulink  SourceProductBaseCode=SL
  Constant : Constant  Value=50
  Constant1 : Constant  Value=9
  Constant2 : Constant  Value=182
  Constant3 : Constant  Value=100
  Logical Operator : Logic  AllPortsSameDT=off  OutDataTypeStr=boolean
  check turn 2 : Outport
  wires:
  Constant/1 -> Check Dynamic Range/1
  Logical Operator/1 -> check turn 2/1
  Constant2/1 -> Check Dynamic Range1/1
  Constant3/1 -> Check Dynamic Range1/2
  Check Dynamic Range/1 -> Logical Operator/1
  X/1 -> Check Dynamic Range/3
  Constant1/1 -> Check Dynamic Range/2
  Check Dynamic Range1/1 -> Logical Operator/2
  Y/1 -> Check Dynamic Range1/3

== system solution1_7009_newfmu/Control Algorithm/Track Segment Identifier/1 if in transition phase ==
  X : Inport
  Y : Inport  Port=2
  Check Dynamic Range : simulink/Model Verification/Check  Dynamic Range  Description=min < u < max  enabled=off  stopWhenAssertionFail=off  export=on  icon=graphic
      settings: SourceProductName=Simulink  SourceProductBaseCode=SL
  Check Dynamic Range1 : simulink/Model Verification/Check  Dynamic Range  Description=min < u < max  enabled=off  stopWhenAssertionFail=off  export=on  icon=graphic
      settings: SourceProductName=Simulink  SourceProductBaseCode=SL
  Constant : Constant  Value=89.5
  Constant1 : Constant  Value=21
  Constant2 : Constant  Value=106
  Constant3 : Constant  Value=89.5
  Logical Operator : Logic  AllPortsSameDT=off  OutDataTypeStr=boolean
  check transition : Outport
  wires:
  Y/1 -> Check Dynamic Range1/3
  Check Dynamic Range1/1 -> Logical Operator/2
  Constant1/1 -> Check Dynamic Range/2
  X/1 -> Check Dynamic Range/3
  Check Dynamic Range/1 -> Logical Operator/1
  Constant3/1 -> Check Dynamic Range1/2
  Constant2/1 -> Check Dynamic Range1/1
  Logical Operator/1 -> check transition/1
  Constant/1 -> Check Dynamic Range/1

== system solution1_7009_newfmu/Control Algorithm/Control/Drift generate/Max wheel force ==
  Fxmax : Inport
  Fymax : Inport  Port=2
  Gain : Gain  Gain=r
  Terminator : Terminator
  Wheel Traction control : Subsystem
  TxRL : Outport
  TxRR : Outport  Port=2
  wires:
  Wheel Traction control/1(cmd_Tx_3) -> TxRL/1  "TxRL"
  Fymax/1 -> Terminator/1
  Gain/1 -> Wheel Traction control/1(Txmargin)
  Fxmax/1 -> Gain/1
  Wheel Traction control/2("cmd_Tx_4 ") -> TxRR/1  "TxRR"

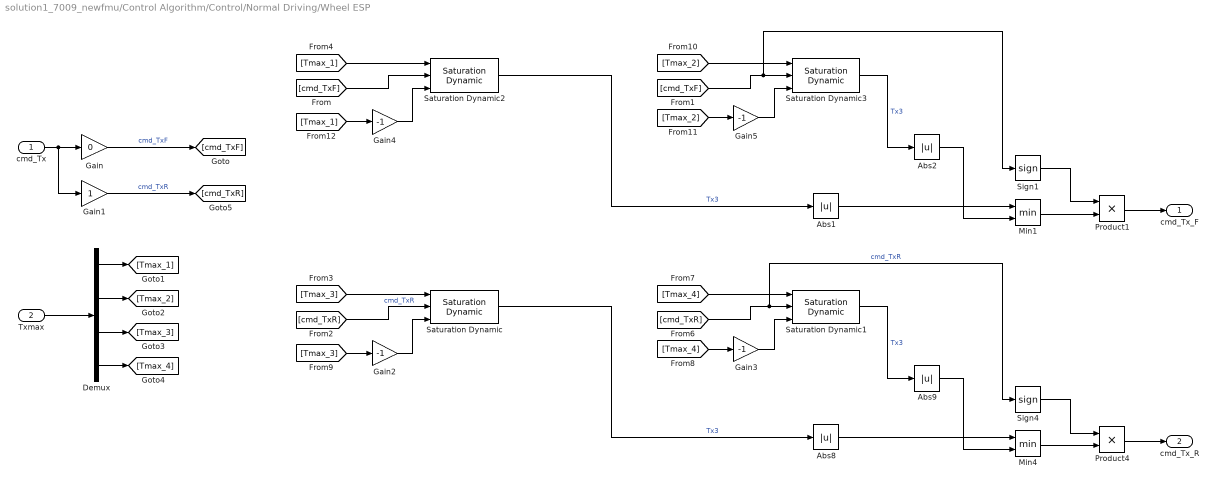
== system solution1_7009_newfmu/Control Algorithm/Control/Normal Driving/Wheel ESP ==
  cmd_Tx : Inport
  Txmax : Inport  Port=2
  Abs{1..2,8..9} (4 alike) : Abs
  Demux : Demux
  Gain : Gain  Gain=0
  Gain1 : Gain
  Gain{2..5} (4 alike) : Gain  Gain=-1
  Min1 : MinMax  Inputs=2
  Min4 : MinMax  Inputs=2
  Product1 : Product
  Product4 : Product
  Saturation Dynamic{,1..3} (4 alike) : simulink/Discontinuities/Saturation Dynamic  OutMin=[]  OutMax=[]  OutDataTypeStr=Inherit: Same as second input  OutDataType=fixdt(1, 16)  OutScaling=2^-10  DoSatur=off
  Sign1 : Signum
  Sign4 : Signum
  cmd_Tx_F : Outport
  cmd_Tx_R : Outport  Port=2
  wires:
  Txmax/1 -> Demux/1
  Demux/1 -> [Tmax_1]
  Demux/2 -> [Tmax_2]
  Demux/3 -> [Tmax_3]
  Demux/4 -> [Tmax_4]
  [cmd_TxR] -> Saturation Dynamic/2  "cmd_TxR"
  [Tmax_3] -> Saturation Dynamic/1
  Saturation Dynamic/1 -> Abs8/1  "Tx3"
  Gain/1 -> [cmd_TxF]  "cmd_TxF"
  cmd_Tx/1 -> Gain1/1, Gain/1
  Gain1/1 -> [cmd_TxR]  "cmd_TxR"
  Abs8/1 -> Min4/1
  Abs9/1 -> Min4/2
  Min4/1 -> Product4/2
  Product4/1 -> cmd_Tx_R/1
  Sign4/1 -> Product4/1
  Gain2/1 -> Saturation Dynamic/3
  [Tmax_4] -> Saturation Dynamic1/1
  [cmd_TxR] -> Sign4/1, Saturation Dynamic1/2  "cmd_TxR"
  Gain3/1 -> Saturation Dynamic1/3
  Saturation Dynamic1/1 -> Abs9/1  "Tx3"
  [Tmax_4] -> Gain3/1
  [Tmax_3] -> Gain2/1
  Abs2/1 -> Min1/2
  Abs1/1 -> Min1/1
  Gain5/1 -> Saturation Dynamic3/3
  [cmd_TxF] -> Sign1/1, Saturation Dynamic3/2
  [Tmax_2] -> Saturation Dynamic3/1
  Saturation Dynamic2/1 -> Abs1/1  "Tx3"
  [Tmax_1] -> Gain4/1
  [cmd_TxF] -> Saturation Dynamic2/2
  [Tmax_1] -> Saturation Dynamic2/1
  Gain4/1 -> Saturation Dynamic2/3
  Product1/1 -> cmd_Tx_F/1
  [Tmax_2] -> Gain5/1
  Min1/1 -> Product1/2
  Sign1/1 -> Product1/1
  Saturation Dynamic3/1 -> Abs2/1  "Tx3"

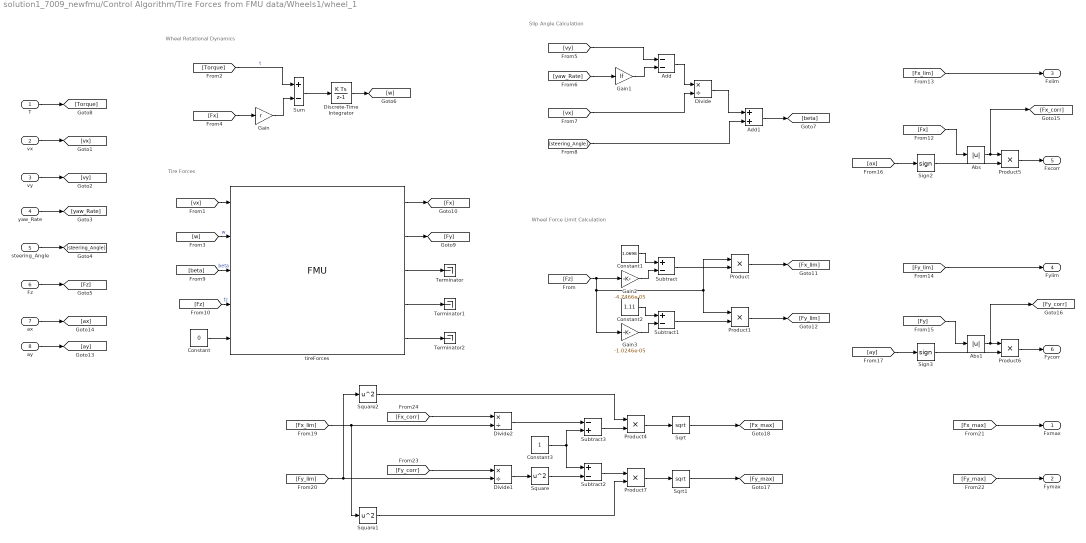
== system solution1_7009_newfmu/Control Algorithm/Tire Forces from FMU data/Wheels1/wheel_1 ==
  note: Wheel Force Limit Calculation
  note: Tire Forces
  note: Wheel Rotational Dynamics
  note: Slip Angle Calculation
  T : Inport
  vx : Inport  Port=2
  vy : Inport  Port=3
  yaw_Rate : Inport  Port=4
  steering_Angle : Inport  Port=5
  Fz : Inport  Port=6
  ax : Inport  Port=7
  ay : Inport  Port=8
  Abs : Abs
  Abs1 : Abs
  Add : Sum  Inputs=--
  Add1 : Sum
  Constant : Constant  Value=0
  Constant1 : Constant  Value=1.0698
  Constant2 : Constant  Value=1.11
  Constant3 : Constant
  Discrete-Time Integrator : DiscreteIntegrator  InitialConditionSetting=State (most efficient)  SampleTime=-1  ICPrevOutput=DiscIntNeverNeededParam  ICPrevScaledInput=DiscIntNeverNeededParam
  Divide : Product  Inputs=*/
  Divide1 : Product  Inputs=*/
  Divide2 : Product  Inputs=*/
  Gain : Gain  Gain=r
  Gain1 : Gain  Gain=lf
  Gain2 : Gain  Gain=-4.7466e-05
  Gain3 : Gain  Gain=-1.0246e-05
  Product{,1,4..7} (6 alike) : Product
  Sign2 : Signum
  Sign3 : Signum
  Sqrt : Sqrt  SaturateOnIntegerOverflow=on
  Sqrt1 : Sqrt  SaturateOnIntegerOverflow=on
  Square : Math  Operator=square  RndMeth=Zero  SaturateOnIntegerOverflow=on
  Square1 : Math  Operator=square  RndMeth=Zero  SaturateOnIntegerOverflow=on
  Square2 : Math  Operator=square  RndMeth=Zero  SaturateOnIntegerOverflow=on
  Subtract : Sum  Inputs=+-
  Subtract1 : Sum  Inputs=+-
  Subtract2 : Sum  Inputs=+-
  Subtract3 : Sum  Inputs=-+
  Sum : Sum  Inputs=+-
  Terminator : Terminator
  Terminator1 : Terminator
  Terminator2 : Terminator
  tireForces : FMU  FMUName=MED2018_TireModel.fmu  FMUMode=CoSimulation  FMUSampleTime=-1  mask(TyreFMUContainer [Co-Simulation, v2.0]){}
      mask Display:
      | disp('TyreFMUContainer');
      | port_label('output',1,'Fx');
      | port_label('output',2,'Fy');
      | port_label('output',3,'Mz');
      | port_label('output',4,'r');
      | port_label('output',5,'Mx');
      | port_label('input',1,'vx');
      | port_label('input',2,'w');
      | port_label('input',3,'beta');
      | port_label('input',4,'Fz');
      | port_label('input',5,'camber');
  Fxmax : Outport
  Fymax : Outport  Port=2
  Fxlim : Outport  Port=3
  Fylim : Outport  Port=4
  Fxcorr : Outport  Port=5
  Fycorr : Outport  Port=6
  wires:
  Discrete-Time Integrator/1 -> [w]
  tireForces/5 -> Terminator2/1
  tireForces/2 -> [Fy]
  tireForces/4 -> Terminator1/1
  tireForces/3 -> Terminator/1
  Sum/1 -> Discrete-Time Integrator/1
  [Torque] -> Sum/1  "t"
  Gain/1 -> Sum/2
  [Fx] -> Gain/1
  Constant/1 -> tireForces/5
  Gain1/1 -> Add/2
  Add/1 -> Divide/1
  [w] -> tireForces/2  "w"
  vx/1 -> [vx]
  vy/1 -> [vy]
  steering_Angle/1 -> [steering_Angle]
  yaw_Rate/1 -> [yaw_Rate]
  Fz/1 -> [Fz]
  [vx] -> tireForces/1
  [vy] -> Add/1
  [yaw_Rate] -> Gain1/1
  [vx] -> Divide/2
  Divide/1 -> Add1/1
  [steering_Angle] -> Add1/2
  Add1/1 -> [beta]
  [beta] -> tireForces/3  "beta"
  [Fz] -> tireForces/4  "fz"
  T/1 -> [Torque]
  tireForces/1 -> [Fx]
  Subtract/1 -> Product/2
  Product/1 -> [Fx_lim]
  Constant2/1 -> Subtract1/1
  Product1/1 -> [Fy_lim]
  Constant1/1 -> Subtract/1
  Gain3/1 -> Subtract1/2
  [Fz] -> Gain3/1, Product/1, Product1/1, Gain2/1
  Subtract1/1 -> Product1/2
  Gain2/1 -> Subtract/2
  Abs1/1 -> [Fy_corr], Product6/1
  [Fx_lim] -> Fxlim/1
  ay/1 -> [ay]
  [Fx] -> Abs/1
  [Fy] -> Abs1/1
  Abs/1 -> [Fx_corr], Product5/1
  Sign2/1 -> Product5/2
  [ax] -> Sign2/1
  [Fy_lim] -> Fylim/1
  [ay] -> Sign3/1
  ax/1 -> [ax]
  Sign3/1 -> Product6/2
  Product5/1 -> Fxcorr/1
  Product6/1 -> Fycorr/1
  [Fy_corr] -> Divide1/1
  [Fy_lim] -> Divide1/2, Square2/1
  [Fx_lim] -> Divide2/2, Square1/1
  [Fx_corr] -> Divide2/1
  Divide1/1 -> Square/1
  Square/1 -> Subtract2/2
  Constant3/1 -> Subtract3/2, Subtract2/1
  Divide2/1 -> Subtract3/1
  Subtract3/1 -> Product4/2
  Subtract2/1 -> Product7/1
  Square1/1 -> Product7/2
  Square2/1 -> Product4/1
  Product7/1 -> Sqrt1/1
  Product4/1 -> Sqrt/1
  Sqrt1/1 -> [Fy_max]
  Sqrt/1 -> [Fx_max]
  [Fx_max] -> Fxmax/1
  [Fy_max] -> Fymax/1
